simulink model "simulaciones_acciones"  (R2020b)
settings: Solver=VariableStepAuto  StartTime=0.0  StopTime=10  RelTol=1e-3
values from neighbouring files (symbols this model uses):
  k = 1    [simualciones_ac.m]
  Kp = 7    [simualciones_ac.m]
  tao = 1    [simualciones_ac.m]
  Td = 1    [simualciones_ac.m]
  Ti = 1    [simualciones_ac.m]
libraries: pid_lib x2
settings Model: Creator=Acer  LastModifiedBy=Acer

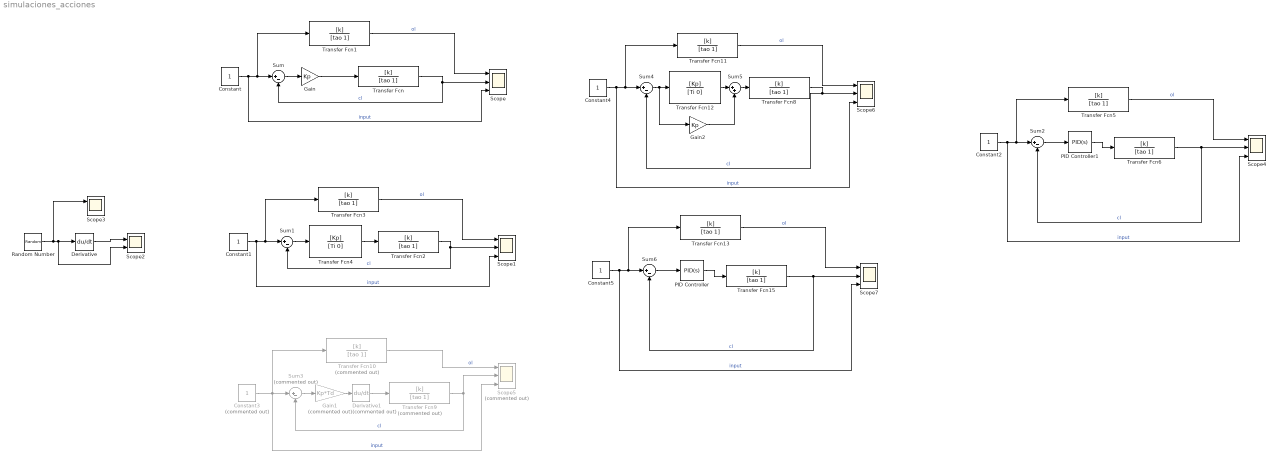
== system simulaciones_acciones ==
  Constant{,1..2,4..5} (5 alike) : Constant
  Constant3 : Constant  Commented=on
  Derivative : Derivative  CoefficientInTFapproximation=0
  Derivative1 : Derivative  Commented=on  CoefficientInTFapproximation=0
  Gain : Gain  Gain=Kp
  Gain1 : Gain  Commented=on  Gain=Kp*Td
  Gain2 : Gain  Gain=Kp
  PID Controller : pid_lib/PID Controller  Controller=PID  Form=Parallel  TimeDomain=Continuous-time  UseExternalTs=off  SampleTime=-1  IntegratorMethod=Forward Euler  FilterMethod=Forward Euler  ControllerParametersSource=internal  P=Kp  I=0  D=Kp*Td  UseFilter=on  N=100  TunerSelectOption=Transfer Function Based (PID Tuner App)  InitialConditionSource=internal  InitialConditionForIntegrator=0  InitialConditionForFilter=0  DifferentiatorICPrevScaledInput=0  ExternalReset=none  TrackingMode=off  Kt=1  LimitOutput=off  SatLimitsSource=internal  UpperSaturationLimit=inf  LowerSaturationLimit=-inf  LinearizeAsGain=on  AntiWindupMode=none  Kb=1  POutMin=[]  POutMax=[]  IOutMin=[]  IOutMax=[]  DOutMin=[]  DOutMax=[]  NOutMin=[]  NOutMax=[]  SumOutMin=[]  SumOutMax=[]  SaturationOutMin=[]  SaturationOutMax=[]  PParamMin=[]  PParamMax=[]  IParamMin=[]  IParamMax=[]  DParamMin=[]  DParamMax=[]  NParamMin=[]  NParamMax=[]  KbParamMin=[]  KbParamMax=[]  KtParamMin=[]  KtParamMax=[]  KbOutMin=[]  KbOutMax=[]  KtOutMin=[]  KtOutMax=[]  IntegratorOutMin=[]  IntegratorOutMax=[]  FilterOutMin=[]  FilterOutMax=[]  SumI1OutMin=[]  SumI1OutMax=[]  SumI2OutMin=[]  SumI2OutMax=[]  SumI3OutMin=[]  SumI3OutMax=[]  SumI4OutMin=[]  SumI4OutMax=[]  SumDOutMin=[]  SumDOutMax=[]  DifferentiatorOutMin=[]  DifferentiatorOutMax=[]  FilterDiffOutCoefMin=[]  FilterDiffOutCoefMax=[]  ReciprocalOutMin=[]  ReciprocalOutMax=[]  SumDenOutMin=[]  SumDenOutMax=[]  SumNumOutMin=[]  SumNumOutMax=[]  DivideOutMin=[]  DivideOutMax=[]  UdiffTsProdOutMin=[]  UdiffTsProdOutMax=[]  NTsProdOutMin=[]  NTsProdOutMax=[]  UintegralTsProdOutMin=[]  UintegralTsProdOutMax=[]  UngainTsProdOutMin=[]  UngainTsProdOutMax=[]  IntegratorContinuousStateAttributes=''  IntegratorStateMustResolveToSignalObject=off  IntegratorRTWStateStorageClass=Auto  FilterContinuousStateAttributes=''  FilterStateMustResolveToSignalObject=off  FilterRTWStateStorageClass=Auto  ParallelPVariant=InternalParameters  IdealPVariant=Disabled  IVariant=InternalParameters  DVariant=InternalParameters  IntegratorVariant=Continuous  SatVariant=Disabled  AWVariant=Passthrough  PCopyVariant=Disabled  TRVariant=Disabled  FdbkBlocksVariant=Forward  IdealPFdbkVariant=Disabled  SatFdbkVariant=Disabled  DerivativeFilterVariant=ContFilter  NVariant=InternalParameters  NCopyVariant=Disabled  FilterICVariant=InternalICsFilter  IntegratorICVariant=InternalICs  ExternalResetVariant=Disabled  TRSumVariant=Passthrough  SumFdbkVariant=Disabled  SumVariant=Sum_PID  TsampFilterVariant=InternalTs  TsampNgainVariant=Passthrough  TsampIntegralVariant=Passthrough  ExternalSaturationOutDataTypeStr=Inherit: Same as second input
  PID Controller1 : pid_lib/PID Controller  Controller=PID  Form=Parallel  TimeDomain=Continuous-time  UseExternalTs=off  SampleTime=-1  IntegratorMethod=Forward Euler  FilterMethod=Forward Euler  ControllerParametersSource=internal  P=Kp  I=Kp/Ti  D=Kp*Td  UseFilter=on  N=100  TunerSelectOption=Transfer Function Based (PID Tuner App)  InitialConditionSource=internal  InitialConditionForIntegrator=0  InitialConditionForFilter=0  DifferentiatorICPrevScaledInput=0  ExternalReset=none  TrackingMode=off  Kt=1  LimitOutput=off  SatLimitsSource=internal  UpperSaturationLimit=inf  LowerSaturationLimit=-inf  LinearizeAsGain=on  AntiWindupMode=none  Kb=1  POutMin=[]  POutMax=[]  IOutMin=[]  IOutMax=[]  DOutMin=[]  DOutMax=[]  NOutMin=[]  NOutMax=[]  SumOutMin=[]  SumOutMax=[]  SaturationOutMin=[]  SaturationOutMax=[]  PParamMin=[]  PParamMax=[]  IParamMin=[]  IParamMax=[]  DParamMin=[]  DParamMax=[]  NParamMin=[]  NParamMax=[]  KbParamMin=[]  KbParamMax=[]  KtParamMin=[]  KtParamMax=[]  KbOutMin=[]  KbOutMax=[]  KtOutMin=[]  KtOutMax=[]  IntegratorOutMin=[]  IntegratorOutMax=[]  FilterOutMin=[]  FilterOutMax=[]  SumI1OutMin=[]  SumI1OutMax=[]  SumI2OutMin=[]  SumI2OutMax=[]  SumI3OutMin=[]  SumI3OutMax=[]  SumI4OutMin=[]  SumI4OutMax=[]  SumDOutMin=[]  SumDOutMax=[]  DifferentiatorOutMin=[]  DifferentiatorOutMax=[]  FilterDiffOutCoefMin=[]  FilterDiffOutCoefMax=[]  ReciprocalOutMin=[]  ReciprocalOutMax=[]  SumDenOutMin=[]  SumDenOutMax=[]  SumNumOutMin=[]  SumNumOutMax=[]  DivideOutMin=[]  DivideOutMax=[]  UdiffTsProdOutMin=[]  UdiffTsProdOutMax=[]  NTsProdOutMin=[]  NTsProdOutMax=[]  UintegralTsProdOutMin=[]  UintegralTsProdOutMax=[]  UngainTsProdOutMin=[]  UngainTsProdOutMax=[]  IntegratorContinuousStateAttributes=''  IntegratorStateMustResolveToSignalObject=off  IntegratorRTWStateStorageClass=Auto  FilterContinuousStateAttributes=''  FilterStateMustResolveToSignalObject=off  FilterRTWStateStorageClass=Auto  ParallelPVariant=InternalParameters  IdealPVariant=Disabled  IVariant=InternalParameters  DVariant=InternalParameters  IntegratorVariant=Continuous  SatVariant=Disabled  AWVariant=Passthrough  PCopyVariant=Disabled  TRVariant=Disabled  FdbkBlocksVariant=Forward  IdealPFdbkVariant=Disabled  SatFdbkVariant=Disabled  DerivativeFilterVariant=ContFilter  NVariant=InternalParameters  NCopyVariant=Disabled  FilterICVariant=InternalICsFilter  IntegratorICVariant=InternalICs  ExternalResetVariant=Disabled  TRSumVariant=Passthrough  SumFdbkVariant=Disabled  SumVariant=Sum_PID  TsampFilterVariant=InternalTs  TsampNgainVariant=Passthrough  TsampIntegralVariant=Passthrough  ExternalSaturationOutDataTypeStr=Inherit: Same as second input
  Random Number : RandomNumber  Variance=0.1  SampleTime=0.1
  Scope{,1,4,6..7} (5 alike) : Scope  NumInputPorts=3
  Scope2 : Scope  NumInputPorts=2
  Scope3 : Scope  NumInputPorts=2
  Scope5 : Scope  Commented=on  NumInputPorts=3
  Sum{,1..2,4,6} (5 alike) : Sum  Inputs=|+-
  Sum3 : Sum  Commented=on  Inputs=|+-
  Sum5 : Sum  Inputs=|++
  Transfer Fcn{,1..3,5..6,8,11,13,15} (10 alike) : TransferFcn  Numerator=[k]  Denominator=[tao 1]
  Transfer Fcn10 : TransferFcn  Commented=on  Numerator=[k]  Denominator=[tao 1]
  Transfer Fcn12 : TransferFcn  Numerator=[Kp]  Denominator=[Ti 0]
  Transfer Fcn4 : TransferFcn  Numerator=[Kp]  Denominator=[Ti 0]
  Transfer Fcn9 : TransferFcn  Commented=on  Numerator=[k]  Denominator=[tao 1]
  wires:
  Constant/1 -> Scope/3, Transfer Fcn1/1, Sum/1  "input"
  Sum/1 -> Gain/1
  Gain/1 -> Transfer Fcn/1
  Transfer Fcn/1 -> Sum/2, Scope/2  "cl"
  Transfer Fcn1/1 -> Scope/1  "ol"
  Sum1/1 -> Transfer Fcn4/1
  Constant1/1 -> Scope1/3, Transfer Fcn3/1, Sum1/1  "input"
  Transfer Fcn2/1 -> Sum1/2, Scope1/2  "cl"
  Transfer Fcn4/1 -> Transfer Fcn2/1
  Transfer Fcn3/1 -> Scope1/1  "ol"
  Random Number/1 -> Scope3/1, Scope2/2, Derivative/1
  Derivative/1 -> Scope2/1
  Sum3/1 -> Gain1/1
  Derivative1/1 -> Transfer Fcn9/1
  Constant3/1 -> Scope5/3, Sum3/1, Transfer Fcn10/1  "input"
  Transfer Fcn9/1 -> Sum3/2, Scope5/2  "cl"
  Transfer Fcn10/1 -> Scope5/1  "ol"
  Gain1/1 -> Derivative1/1
  Constant4/1 -> Scope6/3, Transfer Fcn11/1, Sum4/1  "input"
  Transfer Fcn11/1 -> Scope6/1  "ol"
  Sum4/1 -> Gain2/1, Transfer Fcn12/1
  Transfer Fcn8/1 -> Sum4/2, Scope6/2  "cl"
  Transfer Fcn12/1 -> Sum5/1
  Sum5/1 -> Transfer Fcn8/1
  Gain2/1 -> Sum5/2
  Sum6/1 -> PID Controller/1
  Transfer Fcn15/1 -> Scope7/2, Sum6/2  "cl"
  Constant5/1 -> Scope7/3, Transfer Fcn13/1, Sum6/1  "input"
  Transfer Fcn13/1 -> Scope7/1  "ol"
  PID Controller/1 -> Transfer Fcn15/1
  Transfer Fcn5/1 -> Scope4/1  "ol"
  Constant2/1 -> Scope4/3, Transfer Fcn5/1, Sum2/1  "input"
  Transfer Fcn6/1 -> Scope4/2, Sum2/2  "cl"
  PID Controller1/1 -> Transfer Fcn6/1
  Sum2/1 -> PID Controller1/1
